simulink model "s06_sig_template"  (R2026a)
settings: Solver=ode4  StopTime=inf  FixedStep=P_sim_dt  EnableMultiTasking=on
InitFcn:
  | s06_data;
values from neighbouring files (symbols this model uses):
  P_c_locate_problist = ones(P_car_cnt, 1, 'single')    [s06_data.m]
  P_display_dt = 50e-3    (= 0.05)    [s06_data.m]
  P_dt = 25e-3    (= 0.025)    [s06_data.m]
  P_p_Bf = 0.7    [d01_data.m]
  P_p_Br = 0.7    [d01_data.m]
  P_p_Cf = 2    [d01_data.m]
  P_p_Cr = 2    [d01_data.m]
  P_p_delta_max = 21.58/180*pi    (= 0.37664205258)    [d01_data.m]    (also in d71_data.m = 0.383972435439)
  P_p_deltan_max = 1    [d01_data.m]    (also in d71_data.m = 0.93)
  P_p_deltan_min = -P_p_deltan_max    (= -1)    [d01_data.m]    (also in d71_data.m = -0.93)
  P_p_Df = 2    [d01_data.m]
  P_p_Dr = 2.5    [d01_data.m]
  P_p_Ef = -0.1    [d01_data.m]
  P_p_EG = 0    [d01_data.m]    (also in d71_data.m = 0.02)
  P_p_Er = -0.05    [d01_data.m]
  P_p_J = 192e-6    (= 0.000192)    [d01_data.m]    (also in d71_data.m = 3e-06)
  P_p_k = 2.51    [d01_data.m]    (also in d71_data.m = 3.4)
  P_p_kd0 = 0.04    [d71_data.m]
  P_p_kd1 = 0.15    [d71_data.m]
  P_p_l = abs(P_p_frontaxle_1 + P_p_rearaxle_1)    [d01_data.m]    (also in d71_data.m = 0.0325)
  P_p_lf = P_p_frontaxle_1    (= 0.05)    [d01_data.m]    (also in d71_data.m = 0.01625)
  P_p_lr = P_p_rearaxle_1    (= 0.049)    [d01_data.m]    (also in d71_data.m = 0.01625)
  P_p_m = 132e-3    (= 0.132)    [d01_data.m]    (also in d71_data.m = 0.013)
  P_p_T = 316e-3    (= 0.316)    [d01_data.m]    (also in d71_data.m = 0.12)
  P_p_Tt = P_p_uTt + P_p_output_Tt    (= 0.11)    [d01_data.m]    (also in d71_data.m = 0.1)
  P_p_un_max = 1    [d01_data.m]    (also in d71_data.m = 0.2)
  P_p_un_min = -P_p_un_max    (= -1)    [d01_data.m]    (also in d71_data.m = -0.2)
  P_p_xvec0 = [ P_p_v0; P_p_s10; P_p_s20; P_p_psi0; 0; 0; 0 ]    [d01_data.m]    (also in d71_data.m)
  P_p_xvec1 = [ P_p_v0; P_p_s11; P_p_s21; P_p_psi1; 0; 0; 0 ]    [d01_data.m]    (also in d71_data.m)
  P_vfilter = single([ 0.0 0.0 ... (first row only)    [s06_data.m]
undefined symbols (not defined in the file or in its folder): CarInputsCmdForward, ManeuverTypePark, ManeuverTypePathFollow, mbc_car_display, P_cpseq, P_p, P_track
libraries: vrlib x2
(part 2 of 2)

== matlab function s06_sig_template/Car0/Motion Control/MPC ==
  data: states input; pedal output; spline input; delta output
function [pedal, delta] = MPC(states, spline)

    N  = 20;
    nd = 4;      % 100 ms / 25 ms

    coder.extrinsic('mpc_step_external');

    %% ================================================================
    % Warm start
    persistent u_warm

    if isempty(u_warm)
        u_warm = zeros(2*N,1);
    else
        % Shift control sequence by one MPC step
        u_warm(1:end-2) = u_warm(3:end);

        % Last pair remains unchanged:
        % effectively repeat final predicted input.
    end


    %% ================================================================
    % Previously issued command
    persistent u_last

    if isempty(u_last)
        u_last = zeros(2,1);
    end


    %% ================================================================
    % Input delay queue
    %
    % columns:
    % [oldest ---------------------- newest]
    %
    % [u_{k-4}, u_{k-3}, u_{k-2}, u_{k-1}]
    %
    persistent u_delay

    if isempty(u_delay)
        u_delay = zeros(2,nd);
    end


    %% ================================================================
    % Solve NMPC

    u_opt = zeros(2*N,1);

    u_opt = mpc_step_external( ...
        states, ...
        u_warm, ...
        u_last, ...
        u_delay, ...
        spline);


    %% First newly commanded input
    u_cmd = u_opt(1:2);

    pedal = u_cmd(1);
    delta = u_cmd(2);


    %% ================================================================
    % Update warm start

    u_warm = u_opt;


    %% ================================================================
    % Update command history

    u_last = u_cmd;


    %% ================================================================
    % Update delay queue

    u_delay(:,1:end-1) = u_delay(:,2:end);
    u_delay(:,end)     = u_cmd;

end

== matlab function s06_sig_template/Car0/Motion Control/MATLAB Function1 ==
  data: sc2e input; psiError input; currentOK output; runOK output; un input; deltan input; lapDone input; reset input; runSuccessful output; trackOK output; inputRateOK output; maxAbsSc2e output; maxAbsPsiError output; maxAbsDun output; maxAbsDdeltan output; P_dt parameter; pedalEffortLast output; steeringEffortLast output
function [currentOK, runOK, runSuccessful, ...
          trackOK, inputRateOK, ...
          maxAbsSc2e, maxAbsPsiError, ...
          maxAbsDun, maxAbsDdeltan, ...
          pedalEffortLast, steeringEffortLast] = ...
    limit_check(sc2e, psiError, un, deltan, ...
                lapDone, reset, P_dt)
% LIMIT_CHECK
%
% Boolean convention:
%   1 = criterion satisfied
%   0 = criterion violated
%
% Inputs
%   sc2e      : signed lateral error [m]
%   psiError  : wrapped heading error [rad]
%   un        : normalized pedal command
%   deltan    : normalized steering command
%   lapDone   : one-sample pulse when one lap is completed
%   reset     : reset monitor
%   P_dt      : sample time [s]
%
% Outputs
%   currentOK          : current sample satisfies all checked limits
%   runOK              : no checked limit has been violated so far
%   runSuccessful      : completed lap with no checked violation
%   trackOK            : track boundary never violated
%   inputRateOK        : actuator rates never violated limits
%   maxAbsSc2e         : maximum absolute lateral error [m]
%   maxAbsPsiError     : maximum absolute heading error [rad]
%   maxAbsDun          : maximum pedal-command rate [1/s]
%   maxAbsDdeltan      : maximum steering-command rate [1/s]
%   pedalEffortLast    : integral of un^2 over last lap
%   steeringEffortLast : integral of deltan^2 over last lap

%% Limits
sc2eMax = 0.06;       % [m]

% Maximum normalized pedal-command rate
dunMax = 3.744;       % [1/s]

% Assumed physical steering speed:
% 3 rev/s = 6*pi rad/s
deltaMaxPhysical  = 0.3839;  % [rad]
ddeltaMaxPhysical = 6*pi;    % [rad/s]

% Convert physical steering rate to normalized steering-command rate
ddeltanMax = ddeltaMaxPhysical * 0.93 / deltaMaxPhysical;

% Numerical tolerance
tol = 1e-9;

%% Persistent states
persistent initialized
persistent previousUn
persistent previousDeltan

persistent trackOKStored
persistent inputRateOKStored

persistent lapCompletedStored
persistent runSuccessfulStored

persistent maxSc2eStored
persistent maxPsiErrorStored
persistent maxDunStored
persistent maxDdeltanStored

persistent pedalEffortAccumulated
persistent steeringEffortAccumulated
persistent savedPedalEffort
persistent savedSteeringEffort

%% Initialize or reset
if isempty(initialized) || reset
    initialized = true;

    previousUn     = double(un);
    previousDeltan = double(deltan);

    trackOKStored     = true;
    inputRateOKStored = true;

    lapCompletedStored  = false;
    runSuccessfulStored = false;

    maxSc2eStored     = abs(double(sc2e));
    maxPsiErrorStored = abs(double(psiError));
    maxDunStored      = 0.0;
    maxDdeltanStored  = 0.0;

    pedalEffortAccumulated    = 0.0;
    steeringEffortAccumulated = 0.0;

    savedPedalEffort    = 0.0;
    savedSteeringEffort = 0.0;

    currentOK     = true;
    runOK         = true;
    runSuccessful = false;

    trackOK     = true;
    inputRateOK = true;

    maxAbsSc2e          = maxSc2eStored;
    maxAbsPsiError      = maxPsiErrorStored;
    maxAbsDun           = maxDunStored;
    maxAbsDdeltan       = maxDdeltanStored;
    pedalEffortLast     = savedPedalEffort;
    steeringEffortLast  = savedSteeringEffort;

    return;
end

%% Calculate actuator rates
if P_dt > 0
    dt = double(P_dt);

    dun = ...
        (double(un) - previousUn) / dt;

    ddeltan = ...
        (double(deltan) - previousDeltan) / dt;
else
    dt = 0.0;

    dun     = inf;
    ddeltan = inf;
end

%% Current-sample checks
trackOKNow = ...
    abs(double(sc2e)) <= sc2eMax + tol;

inputRateOKNow = ...
    abs(dun)     <= dunMax     + tol && ...
    abs(ddeltan) <= ddeltanMax + tol;

currentOK = ...
    trackOKNow && inputRateOKNow;

%% Latch failures
trackOKStored = ...
    trackOKStored && trackOKNow;

inputRateOKStored = ...
    inputRateOKStored && inputRateOKNow;

%% Update maximum observed quantities
maxSc2eStored = max( ...
    maxSc2eStored, ...
    abs(double(sc2e)));

maxPsiErrorStored = max( ...
    maxPsiErrorStored, ...
    abs(double(psiError)));

maxDunStored = max( ...
    maxDunStored, ...
    abs(dun));

maxDdeltanStored = max( ...
    maxDdeltanStored, ...
    abs(ddeltan));

%% Accumulate quadratic control effort
if dt > 0
    pedalEffortAccumulated = ...
        pedalEffortAccumulated + double(un)^2 * dt;

    steeringEffortAccumulated = ...
        steeringEffortAccumulated + double(deltan)^2 * dt;
end

%% Overall run condition
runOK = ...
    trackOKStored && inputRateOKStored;

%% Detect lap completion
if lapDone
    lapCompletedStored  = true;
    runSuccessfulStored = runOK;

    savedPedalEffort = ...
        pedalEffortAccumulated;

    savedSteeringEffort = ...
        steeringEffortAccumulated;

    pedalEffortAccumulated    = 0.0;
    steeringEffortAccumulated = 0.0;
end

runSuccessful = ...
    lapCompletedStored && runSuccessfulStored;

%% Update previous values
previousUn     = double(un);
previousDeltan = double(deltan);

%% Outputs
trackOK     = trackOKStored;
inputRateOK = inputRateOKStored;

maxAbsSc2e         = maxSc2eStored;
maxAbsPsiError     = maxPsiErrorStored;
maxAbsDun          = maxDunStored;
maxAbsDdeltan      = maxDdeltanStored;
pedalEffortLast    = savedPedalEffort;
steeringEffortLast = savedSteeringEffort;

end

== matlab function s06_sig_template/Localization/Locate/ObsSpline/Reference and Deviations ==
  data: wxe output; s input; psi input; widxkm1 input int32; spline input; P_c_spline_range parameter; wx output; ws output; wkappa output; widx output; ey output; epsi output
function [ wxe, wx, ws, wkappa, widx, ey, epsi ] = fcn(s, psi, widxkm1, spline, P_c_spline_range)

wxe = spline.points(1, spline.breakslen);
if widxkm1 < int32(1)
    % first call
    irangemin = int32(1);
    irangemax = int32(spline.breakslen);
else
    irangemin = widxkm1 - P_c_spline_range;
    irangemax = widxkm1 + P_c_spline_range;
end
[ w , widx ] = mbc_spline_get_reference(s, spline.breakslen, spline.points, spline.coefs, spline.periodic, 0, 0, irangemin, irangemax);
wx = w(1);
wpsi = w(2);
ws = w(3:4);
wkappa = w(5);
ey = -sin(wpsi) * (s(1) - ws(1)) + cos(wpsi) * (s(2) - ws(2));
epsi = mod(psi - wpsi + pi, 2*pi) - pi;
end

== matlab function s06_sig_template/Maneuver1/Create Maneuver ==
  data: type input; vmax input; xref input; P_track parameter; P_cpseq parameter; maneuver output Bus: DRIVEMANEUVER size=1
function maneuver = create_maneuver(type, vmax, xref, P_track, P_cpseq)


track = P_track.center;

maneuver = struct( ...
    'vmax', vmax, ... 
    'type', type, ...
    'xref', xref, ...
    'lapCount', uint32(0), ...
    'disableLaneMonitor', false, ...
    'isnew', true, ...
    'breakslen', track.breakslen, ...
    'points', track.points, ...
    'coefs', track.coefs, ...
    'segments', zeros(1, length(track.points), 'uint32'), ...
    'periodic', true, ...
    'cpseq', P_cpseq);
end

== matlab function s06_sig_template/Localization/Locate/ObsSpline/wx derivative ==
  data: wx input; wxm1 input; xe input; wxd output; P_dt parameter
function wxd  = wx2wv(wx, wxm1, xe, P_dt)
wxd = single(0);
if wxm1 > -1
    wxd = (mod(wx - wxm1 + 0.5 * xe, xe) - 0.5 * xe) / P_dt;
end
end

== matlab function s06_sig_template/Maneuver0/Create Maneuver ==
  data: type input; vmax input; xref input; P_track parameter; P_cpseq parameter; maneuver output Bus: DRIVEMANEUVER size=1
function maneuver = create_maneuver(type, vmax, xref, P_track, P_cpseq)


track = P_track.center;

maneuver = struct( ...
    'vmax', vmax, ... 
    'type', type, ...
    'xref', xref, ...
    'lapCount', uint32(0), ...
    'disableLaneMonitor', false, ...
    'isnew', true, ...
    'breakslen', track.breakslen, ...
    'points', track.points, ...
    'coefs', track.coefs, ...
    'segments', zeros(1, length(track.points), 'uint32'), ...
    'periodic', true, ...
    'cpseq', P_cpseq);
end

== matlab function s06_sig_template/Localization/Locate/ObsSpline/Reference and Deviations1 ==
  data: wxe output; s input; psi input; widxkm1 input int32; spline input; P_c_spline_range parameter; w output; widx output; ey output; epsi output
function [ wxe, w, widx, ey, epsi ] = fcn(s, psi, widxkm1, spline, P_c_spline_range)

wxe = spline.points(1, spline.breakslen);
if widxkm1 < int32(1)
    % first call
    irangemin = int32(1);
    irangemax = int32(spline.breakslen);
else
    irangemin = widxkm1 - P_c_spline_range;
    irangemax = widxkm1 + P_c_spline_range;
end
[ w , widx ] = mbc_spline_get_reference(s, spline.breakslen, spline.points, spline.coefs, spline.periodic, 0, 0, irangemin, irangemax);
wpsi = w(2);
ws = w(3:4);
ey = -sin(wpsi) * (s(1) - ws(1)) + cos(wpsi) * (s(2) - ws(2));
epsi = mod(psi - wpsi + pi, 2*pi) - pi;
end

== matlab function s06_sig_template/Localization/Locate/ObsSpline/Reference and Deviations2 ==
  data: wxe output; s input; psi input; widxkm1 input int32; spline input; P_c_spline_range parameter; w output; widx output; ey output; epsi output
function [ wxe, w, widx, ey, epsi ] = fcn(s, psi, widxkm1, spline, P_c_spline_range)

wxe = spline.points(1, spline.breakslen);
if widxkm1 < int32(1)
    % first call
    irangemin = int32(1);
    irangemax = int32(spline.breakslen);
else
    irangemin = widxkm1 - P_c_spline_range;
    irangemax = widxkm1 + P_c_spline_range;
end
[ w , widx ] = mbc_spline_get_reference(s, spline.breakslen, spline.points, spline.coefs, spline.periodic, 0, 0, irangemin, irangemax);
wpsi = w(2);
ws = w(3:4);
ey = -sin(wpsi) * (s(1) - ws(1)) + cos(wpsi) * (s(2) - ws(2));
epsi = mod(psi - wpsi + pi, 2*pi) - pi;
end
